simulink model "mass_spring_damper_linear_ADRC"  (R2018b)
settings: Solver=VariableStepAuto  StartTime=0.0  StopTime=30  RelTol=1e-3
PreLoadFcn:
  | AM = 1;
  | TM = 1;
  | O = 0;
  | Am = 1;
  | Tm = 1;
  | frst = 0;
  | scnd = 0;
  | thrd = 0;
  | frth = 0;
  | ffth = 0;
  | t1 = 0;
  | t2 = 0;
  | t3 = 0;
  | t4 = 0;
InitFcn:
  | %%%%%%%%%%%%%%%%%%%%%%%%%
  | %                  TUNABLE PARAMETERS              %
  | %(ORDER, SETTLING TIME, ESO GAIN AND B0)%
  | %%%%%%%%%%%%%%%%%%%%%%%%%
  | order = 2;                  % ADRC order
  | ts = 2;                        % Desired settling time
  | b0 = 1;                       % b0 parameter
  | eso_gain = 10;           % ESO Dynamic related to closed-loop poles
  | 
  | %%%%%%%%%%%%%%%%%%%%%%%%%
  | %                                 ADRC                               %
  | %      (CONTROLLER GAINS AND ESO MATRIXES)    %
  | %%%%%%%%%%%%%%%%%%%%%%%%%
  | s_cl = 4/ts;                           % Closed-loop system poles
  | s_eso = eso_gain * s_cl;        % ESO poles
  | pole = [1 s_cl];                     % Base polynomial to calculate
  |                                            % System characteristic polynomial
  | pole_eso = [1 s_eso];            % Base polynomial to calculate
  |                                            % ESO characteristic polynomial
  | A = zeros(order + 1);            % Matrix A of ESO
  | B = zeros(order + 1, 1);        % Matrix B of ESO
  | C = [1 zeros(1, order)];         % Matrix C of ESO
  | 
  | %%%%%%%%%%%%%%%%%%%%%%%%%%%%%%%%%%%
  | % Here we'll calculate the characteristic polynomials of system and ESO,   %
  | % starting with the base polynomial, and convoluting it until we achieve    %
  | % the system's order.                                                                           %
  | % Also, we'll put the values of A and B matrixes of ESO, filling the             %
  | % diagonal above the main diagonal of A with one's, and putting the value %
  | % b0 on the penultimate value of B matrix, according to ADRC generalized %
  | % model fot Nth order.                                                                          %
  | %%%%%%%%%%%%%%%%%%%%%%%%%%%%%%%%%%%
  | A_sys = pole;
  | A_eso = pole_eso;
  | 
  | for i = 1:order
  |     if i ~= order
  |         A_sys = conv(A_sys, pole);
  |     else
  |         B(i) = b0;
  |     end
  |     A(i,i+1) = 1;
  |     A_eso = conv(A_eso, pole_eso);
  | end
  | 
  | K = [1 A_sys(2:end)];           % Controller gain matrix
  | L = A_eso(2:end)';               % ESO gain matrix
  | 
  | %%%%%%%%%%%%%%%%%%%%%%%%
  | %                  SYSTEM PARAMETERS             %
  | %%%%%%%%%%%%%%%%%%%%%%%%
  | 
  | m1 = 0.3;                       % Mass one value
  | m2 = 1;                     % Mass two value
  | k = 0.8;
  | k2 = 0;                          % Spring constant
  | k3 = 0;
  | fv1 = 0.7;
  | fv2 = 1;
  | b = 1;                          % Friction coefficient
libraries: dspindex x1
settings Model: Creator=root  LastModifiedBy=root

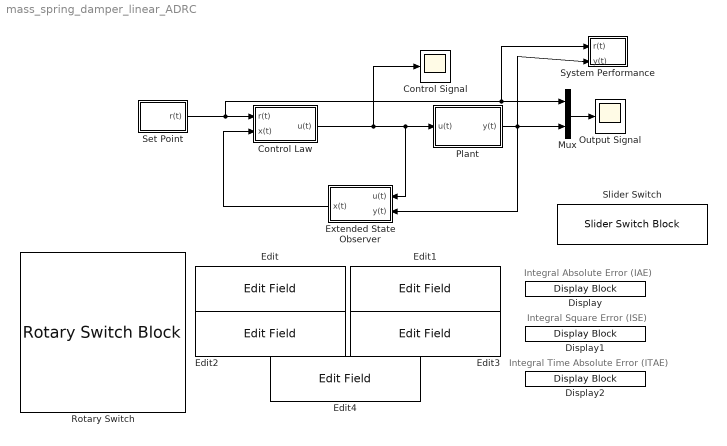
== system mass_spring_damper_linear_ADRC ==
  note: Integral Absolute Error (IAE)
  note: Integral Square Error (ISE)
  note: Integral Time Absolute Error (ITAE)
  Control Law : Subsystem
  Control Signal : Scope
  Display : DisplayBlock  WebBlockId=203  LabelPosition=Hide
  Display1 : DisplayBlock  WebBlockId=209  LabelPosition=Hide
  Display2 : DisplayBlock  WebBlockId=215  LabelPosition=Hide
  Edit : EditField  WebBlockId=70  ShowInitialText=on  Alignment=Center
  Edit1 : EditField  WebBlockId=71  ShowInitialText=on  Alignment=Center
  Edit2 : EditField  WebBlockId=72  ShowInitialText=on  Alignment=Center
  Edit3 : EditField  WebBlockId=73  ShowInitialText=on  Alignment=Center
  Edit4 : EditField  WebBlockId=74  ShowInitialText=on  Alignment=Center
  Extended State Observer : Subsystem
  Mux : Mux  Inputs=2
  Output Signal : Scope
  Plant : Subsystem
  Rotary Switch : RotarySwitchBlock  WebBlockId=122
      settings: Values={{'Step', 'Sine', 'Sawtooth', 'Square', 'Random'}, [0 1 2 3 4]}
  Set Point : Subsystem
  Slider Switch : SliderSwitchBlock  WebBlockId=63
      settings: Values={{'Mass 1', 'Mass 2'}, [1 0]}
  System Performance : Subsystem
  wires:
  Plant/1(y(t)) -> Extended State Observer/2(y(t)), System Performance/2(y(t)), Mux/2
  Control Law/1(u(t)) -> Extended State Observer/1("u(t) "), Plant/1(u(t)), Control Signal/1
  Set Point/1(r(t)) -> Control Law/1(r(t)), Mux/1, System Performance/1(r(t))
  Mux/1 -> Output Signal/1
  Extended State Observer/1(x(t)) -> Control Law/2(x(t))

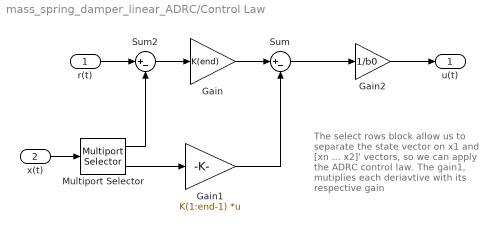
== system mass_spring_damper_linear_ADRC/Control Law ==
  note: The select rows block allow us to separate the state vector on x1 and [xn ... x2]' vectors, so we can apply the ADRC control law. The gain1, mutiplies each deriavtive with its respective gain
  r(t) : Inport
  x(t) : Inport  Port=2
  Gain : Gain  Gain=K(end)  ParamDataTypeStr=Inherit: Inherit from 'Gain'
  Gain1 : Gain  Gain=K(1:end-1)  Multiplication=Matrix(K*u) (u vector)
  Gain2 : Gain  Gain=1/b0
  Multiport Selector : dspindex/Multiport Selector  rowsOrCols=Rows  idxCellArray={ 1, [order+1:-1:2]}  idxErrMode=Clip Index
  Sum : Sum  Inputs=|+-
  Sum2 : Sum  Inputs=|+-
  u(t) : Outport
  wires:
  Gain2/1 -> u(t)/1
  Sum/1 -> Gain2/1
  r(t)/1 -> Sum2/1
  Sum2/1 -> Gain/1
  Gain/1 -> Sum/1
  x(t)/1 -> Multiport Selector/1
  Multiport Selector/1 -> Sum2/2
  Multiport Selector/2 -> Gain1/1
  Gain1/1 -> Sum/2

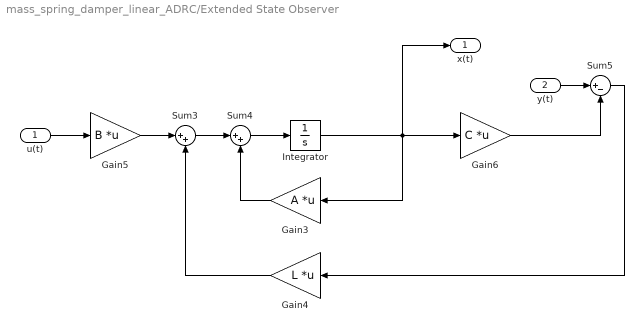
== system mass_spring_damper_linear_ADRC/Extended State Observer ==
  "u(t) " : Inport
  y(t) : Inport  Port=2
  Gain3 : Gain  Gain=A  Multiplication=Matrix(K*u) (u vector)
  Gain4 : Gain  Gain=L  Multiplication=Matrix(K*u) (u vector)
  Gain5 : Gain  Gain=B  Multiplication=Matrix(K*u) (u vector)
  Gain6 : Gain  Gain=C  Multiplication=Matrix(K*u) (u vector)
  Integrator : Integrator
  Sum3 : Sum  Inputs=|++
  Sum4 : Sum  Inputs=|++
  Sum5 : Sum  Inputs=|+-
  x(t) : Outport
  wires:
  Sum4/1 -> Integrator/1
  y(t)/1 -> Sum5/1
  Gain4/1 -> Sum3/2
  Gain5/1 -> Sum3/1
  Gain3/1 -> Sum4/2
  Sum3/1 -> Sum4/1
  Sum5/1 -> Gain4/1
  Gain6/1 -> Sum5/2
  Integrator/1 -> x(t)/1, Gain3/1, Gain6/1
  "u(t) "/1 -> Gain5/1

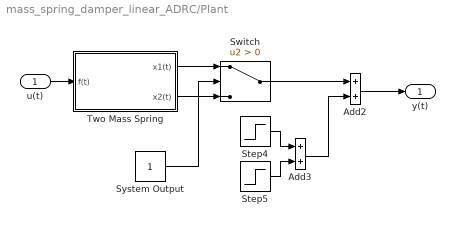
== system mass_spring_damper_linear_ADRC/Plant ==
  u(t) : Inport
  Add2 : Sum
  Add3 : Sum
  Step4 : Step  Time=22  After=-0.5  SampleTime=0
  Step5 : Step  Time=11  After=0.5  SampleTime=0
  Switch : Switch  Criteria=u2 > Threshold
  System Output : Constant
  Two Mass Spring : Subsystem
  y(t) : Outport
  wires:
  u(t)/1 -> Two Mass Spring/1(f(t))
  System Output/1 -> Switch/2
  Two Mass Spring/2(x2(t)) -> Switch/3
  Two Mass Spring/1(x1(t)) -> Switch/1
  Switch/1 -> Add2/1
  Add2/1 -> y(t)/1
  Step4/1 -> Add3/1
  Step5/1 -> Add3/2
  Add3/1 -> Add2/2

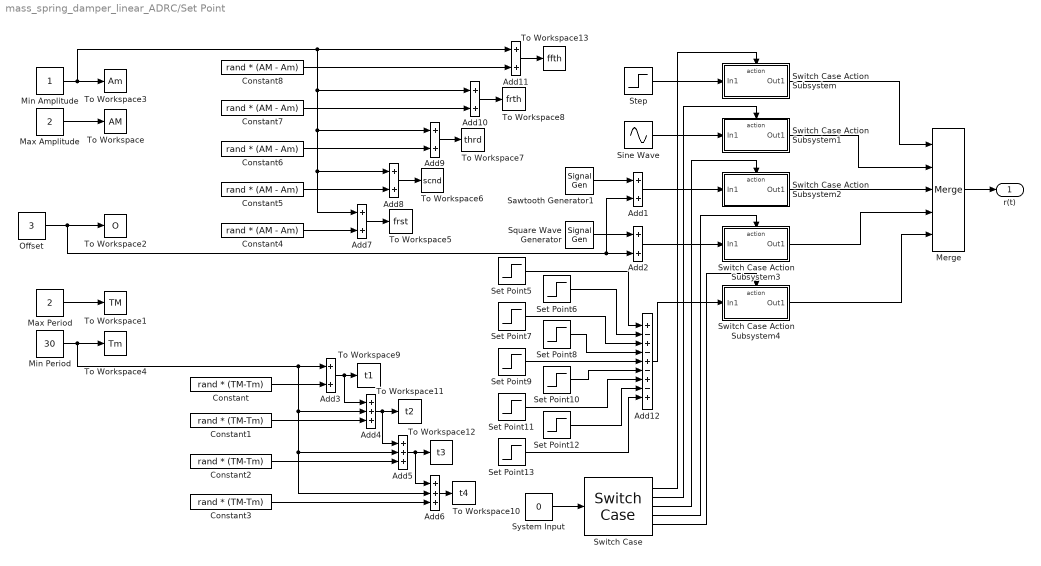
== system mass_spring_damper_linear_ADRC/Set Point ==
  Add{1..3,7} (4 alike) : Sum  Inputs=2
  Add{8..11} (4 alike) : Sum
  Add12 : Sum  Inputs=+-+-+-+-+
  Add4 : Sum  Inputs=3
  Add5 : Sum  Inputs=3
  Add6 : Sum  Inputs=3
  Constant{,1..3} (4 alike) : Constant  Value=rand * (TM-Tm)
  Constant{4..8} (5 alike) : Constant  Value=rand * (AM - Am)
  Max Amplitude : Constant  Value=2  VectorParams1D=off
  Max Period : Constant  Value=2  VectorParams1D=off
  Merge : Merge  Inputs=5
  Min Amplitude : Constant  VectorParams1D=off
  Min Period : Constant  Value=30  VectorParams1D=off
  Offset : Constant  Value=3  VectorParams1D=off
  Sawtooth Generator1 : SignalGenerator  WaveForm=sawtooth  Amplitude=AM  Frequency=1/TM  Units=rad/sec
  Set Point10 : Step  Time=t3  After=thrd  SampleTime=0
  Set Point11 : Step  Time=t3  After=frth  SampleTime=0
  Set Point12 : Step  Time=t4  After=frth  SampleTime=0
  Set Point13 : Step  Time=t4  After=ffth  SampleTime=0
  Set Point5 : Step  Time=0  After=frst  SampleTime=0
  Set Point6 : Step  Time=t1  After=frst  SampleTime=0
  Set Point7 : Step  Time=t1  After=scnd  SampleTime=0
  Set Point8 : Step  Time=t2  After=scnd  SampleTime=0
  Set Point9 : Step  Time=t2  After=thrd  SampleTime=0
  Sine Wave : Sin  Amplitude=AM  Bias=O  Frequency=1/TM  SampleTime=0
  Square Wave Generator : SignalGenerator  WaveForm=square  Amplitude=AM  Frequency=1/TM  Units=rad/sec
  Step : Step  After=AM  SampleTime=0
  Switch Case : SwitchCase  CaseConditions={0,1,2,3,4}  ShowDefaultCase=off
  Switch Case Action Subsystem : Subsystem  TreatAsAtomicUnit=on
  Switch Case Action Subsystem1 : Subsystem  TreatAsAtomicUnit=on
  Switch Case Action Subsystem2 : Subsystem  TreatAsAtomicUnit=on
  Switch Case Action Subsystem3 : Subsystem  TreatAsAtomicUnit=on
  Switch Case Action Subsystem4 : Subsystem  TreatAsAtomicUnit=on
  System Input : Constant  Value=0
  To Workspace : ToWorkspace  VariableName=AM  SampleTime=-1
      settings: MaxDataPoints=1
  To Workspace1 : ToWorkspace  VariableName=TM  SampleTime=-1
      settings: MaxDataPoints=1
  To Workspace10 : ToWorkspace  VariableName=t4  SampleTime=-1
      settings: MaxDataPoints=1
  To Workspace11 : ToWorkspace  VariableName=t2  SampleTime=-1
      settings: MaxDataPoints=1
  To Workspace12 : ToWorkspace  VariableName=t3  SampleTime=-1
      settings: MaxDataPoints=1
  To Workspace13 : ToWorkspace  VariableName=ffth  SampleTime=-1
      settings: MaxDataPoints=1
  To Workspace2 : ToWorkspace  VariableName=O  SampleTime=-1
      settings: MaxDataPoints=1
  To Workspace3 : ToWorkspace  VariableName=Am  SampleTime=-1
      settings: MaxDataPoints=1
  To Workspace4 : ToWorkspace  VariableName=Tm  SampleTime=-1
      settings: MaxDataPoints=1
  To Workspace5 : ToWorkspace  VariableName=frst  SampleTime=-1
      settings: MaxDataPoints=1
  To Workspace6 : ToWorkspace  VariableName=scnd  SampleTime=-1
      settings: MaxDataPoints=1
  To Workspace7 : ToWorkspace  VariableName=thrd  SampleTime=-1
      settings: MaxDataPoints=1
  To Workspace8 : ToWorkspace  VariableName=frth  SampleTime=-1
      settings: MaxDataPoints=1
  To Workspace9 : ToWorkspace  VariableName=t1  SampleTime=-1
      settings: MaxDataPoints=1
  r(t) : Outport
  wires:
  Merge/1 -> r(t)/1
  Switch Case Action Subsystem3/1(Out1) -> Merge/4
  Switch Case/1 -> Switch Case Action Subsystem/Action
  Max Amplitude/1 -> To Workspace/1
  Square Wave Generator/1 -> Add2/1
  Add1/1 -> Switch Case Action Subsystem2/1(In1)
  Step/1 -> Switch Case Action Subsystem/1(In1)
  Switch Case/3 -> Switch Case Action Subsystem2/Action
  Switch Case/4 -> Switch Case Action Subsystem3/Action
  Switch Case/5 -> Switch Case Action Subsystem4/Action
  Switch Case/2 -> Switch Case Action Subsystem1/Action
  Sawtooth Generator1/1 -> Add1/1
  System Input/1 -> Switch Case/1
  Switch Case Action Subsystem/1(Out1) -> Merge/1
  Add2/1 -> Switch Case Action Subsystem3/1(In1)
  Min Amplitude/1 -> To Workspace3/1, Add7/1, Add8/1, Add9/1, Add10/1, Add11/1
  Max Period/1 -> To Workspace1/1
  Offset/1 -> Add1/2, Add2/2, To Workspace2/1
  Switch Case Action Subsystem4/1(Out1) -> Merge/5
  Switch Case Action Subsystem2/1(Out1) -> Merge/3
  Sine Wave/1 -> Switch Case Action Subsystem1/1(In1)
  Switch Case Action Subsystem1/1(Out1) -> Merge/2
  Min Period/1 -> To Workspace4/1, Add6/2, Add5/2, Add4/2, Add3/1
  Add12/1 -> Switch Case Action Subsystem4/1(In1)
  Constant/1 -> Add3/2
  Add3/1 -> Add4/1, To Workspace9/1
  Add4/1 -> Add5/1, To Workspace11/1
  Constant1/1 -> Add4/3
  Constant2/1 -> Add5/3
  Add6/1 -> To Workspace10/1
  Add5/1 -> Add6/1, To Workspace12/1
  Constant3/1 -> Add6/3
  Add8/1 -> To Workspace6/1
  Add10/1 -> To Workspace8/1
  Add9/1 -> To Workspace7/1
  Add7/1 -> To Workspace5/1
  Constant4/1 -> Add7/2
  Constant5/1 -> Add8/2
  Constant6/1 -> Add9/2
  Constant7/1 -> Add10/2
  Add11/1 -> To Workspace13/1
  Constant8/1 -> Add11/2
  Set Point13/1 -> Add12/9
  Set Point11/1 -> Add12/7
  Set Point9/1 -> Add12/5
  Set Point8/1 -> Add12/4
  Set Point5/1 -> Add12/1
  Set Point12/1 -> Add12/8
  Set Point7/1 -> Add12/3
  Set Point10/1 -> Add12/6
  Set Point6/1 -> Add12/2

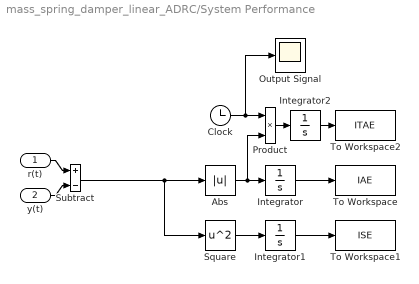
== system mass_spring_damper_linear_ADRC/System Performance ==
  r(t) : Inport
  y(t) : Inport  Port=2
  Abs : Abs
  Clock : Clock
  Integrator : Integrator
  Integrator1 : Integrator
  Integrator2 : Integrator
  Output Signal : Scope
  Product : Product
  Square : Math  Operator=square  SaturateOnIntegerOverflow=on
  Subtract : Sum  Inputs=+-
  To Workspace : ToWorkspace  VariableName=IAE  SaveFormat=Timeseries  SampleTime=-1
  To Workspace1 : ToWorkspace  VariableName=ISE  SaveFormat=Timeseries  SampleTime=-1
  To Workspace2 : ToWorkspace  VariableName=ITAE  SaveFormat=Timeseries  SampleTime=-1
  wires:
  y(t)/1 -> Subtract/2
  r(t)/1 -> Subtract/1
  Abs/1 -> Product/2, Integrator/1
  Subtract/1 -> Square/1, Abs/1
  Integrator/1 -> To Workspace/1
  Integrator1/1 -> To Workspace1/1
  Square/1 -> Integrator1/1
  Clock/1 -> Output Signal/1, Product/1
  Product/1 -> Integrator2/1
  Integrator2/1 -> To Workspace2/1

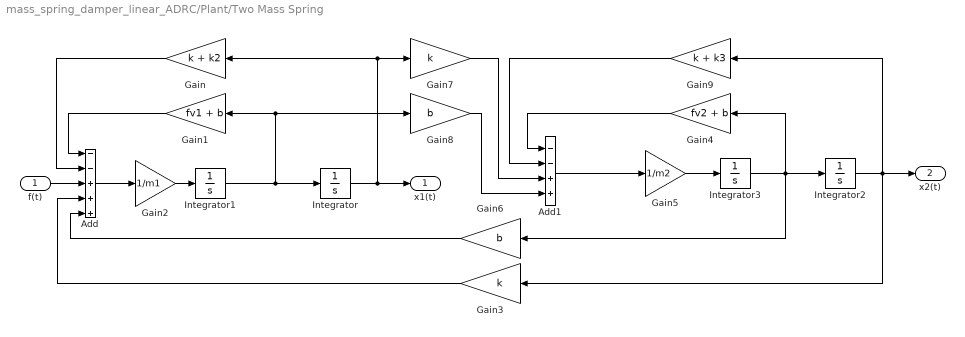
== system mass_spring_damper_linear_ADRC/Plant/Two Mass Spring ==
  f(t) : Inport
  Add : Sum  Inputs=--+++
  Add1 : Sum  Inputs=--++
  Gain : Gain  Gain=k + k2
  Gain1 : Gain  Gain=fv1 + b
  Gain2 : Gain  Gain=1/m1
  Gain3 : Gain  Gain=k
  Gain4 : Gain  Gain=fv2 + b
  Gain5 : Gain  Gain=1/m2
  Gain6 : Gain  Gain=b
  Gain7 : Gain  Gain=k
  Gain8 : Gain  Gain=b
  Gain9 : Gain  Gain=k + k3
  Integrator{,1..3} (4 alike) : Integrator
  x1(t) : Outport
  x2(t) : Outport  Port=2
  wires:
  Integrator/1 -> Gain/1, Gain7/1, x1(t)/1
  Integrator1/1 -> Gain1/1, Gain8/1, Integrator/1
  Integrator3/1 -> Gain6/1, Integrator2/1, Gain4/1
  Gain2/1 -> Integrator1/1
  Add/1 -> Gain2/1
  Add1/1 -> Gain5/1
  Gain5/1 -> Integrator3/1
  f(t)/1 -> Add/3
  Gain1/1 -> Add/1
  Gain/1 -> Add/2
  Gain4/1 -> Add1/1
  Gain3/1 -> Add/4
  Gain6/1 -> Add/5
  Gain7/1 -> Add1/3
  Gain8/1 -> Add1/4
  Gain9/1 -> Add1/2
  Integrator2/1 -> Gain3/1, x2(t)/1, Gain9/1

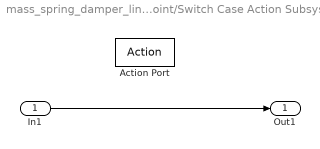
== system mass_spring_damper_linear_ADRC/Set Point/Switch Case Action Subsystem ==
  In1 : Inport
  Action Port : ActionPort  ActionType=case
  Out1 : Outport
  wires:
  In1/1 -> Out1/1

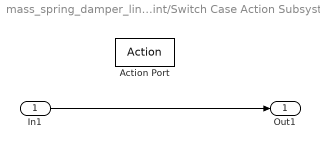
== system mass_spring_damper_linear_ADRC/Set Point/Switch Case Action Subsystem1 ==
  In1 : Inport
  Action Port : ActionPort  ActionType=case
  Out1 : Outport
  wires:
  In1/1 -> Out1/1

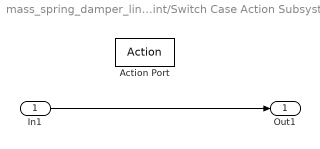
== system mass_spring_damper_linear_ADRC/Set Point/Switch Case Action Subsystem2 ==
  In1 : Inport
  Action Port : ActionPort  ActionType=case
  Out1 : Outport
  wires:
  In1/1 -> Out1/1

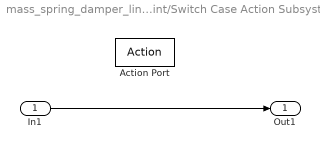
== system mass_spring_damper_linear_ADRC/Set Point/Switch Case Action Subsystem3 ==
  In1 : Inport
  Action Port : ActionPort  ActionType=case
  Out1 : Outport
  wires:
  In1/1 -> Out1/1

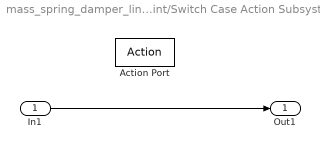
== system mass_spring_damper_linear_ADRC/Set Point/Switch Case Action Subsystem4 ==
  In1 : Inport
  Action Port : ActionPort  ActionType=case
  Out1 : Outport
  wires:
  In1/1 -> Out1/1
